simulink model "SS_continuous_ReducedObs"  (R2021a)
settings: Solver=FixedStepAuto  StartTime=0.0  StopTime=5  FixedStep=0.0001  RelTol=1e-3
values from neighbouring files (symbols this model uses):
  Ao = -1/Tm -Lc    [SS_continuous_ReducedObs_code.m]
  Bo = [km/(gbox.N*Tm), (-1/Tm -Lc)*Lc]    [SS_continuous_ReducedObs_code.m]
  Co = [0;1]    [SS_continuous_ReducedObs_code.m]
  Do = [0, 1; 0, Lc]    [SS_continuous_ReducedObs_code.m]
  K = place(F, G, p)    [SS_allDiscrete_code.m]    (also in SS_continuous_ReducedObs_code.m = place(A, B, p))
  K_robust = [Ked(2), Ked(3)]    [SS_allDiscrete_code.m]    (also in SS_continuous_ReducedObs_code.m = [Ke(2), Ke(3)])
  Ki_robust = Ked(1)    [SS_allDiscrete_code.m]    (also in SS_continuous_ReducedObs_code.m = Ke(1))
  Nu = Nxu(3)    [SS_allDiscrete_code.m]    (also in SS_continuous_ReducedObs_code.m = Nxu(3,3))
  Nx = [Nxu(1); Nxu(2)]    [SS_allDiscrete_code.m]    (also in SS_continuous_ReducedObs_code.m = [Nxu(1,3); Nxu(2,3)])
  rads2rpm = 60/2/pi    (= 9.54929658551)    [load_params_inertial_case.m]
  tauSfEst = 0.0125    [controldesign.m]
  Ts = 0.001    [SS_allDiscrete_code.m]    (also in SS_discrete_ReducedObs_code.m; discretePID_code.m)
undefined symbols (not defined in the file or in its folder): drv, gbox, mld, mot, sens
libraries: simulink x1
settings Model: Creator=giorgiadisaro  LastModifiedBy=utente-A
settings SolverCC: AlgebraicLoopSolver=TrustRegion
settings DebuggingCC: SFMachineParentedDataDiag=warning

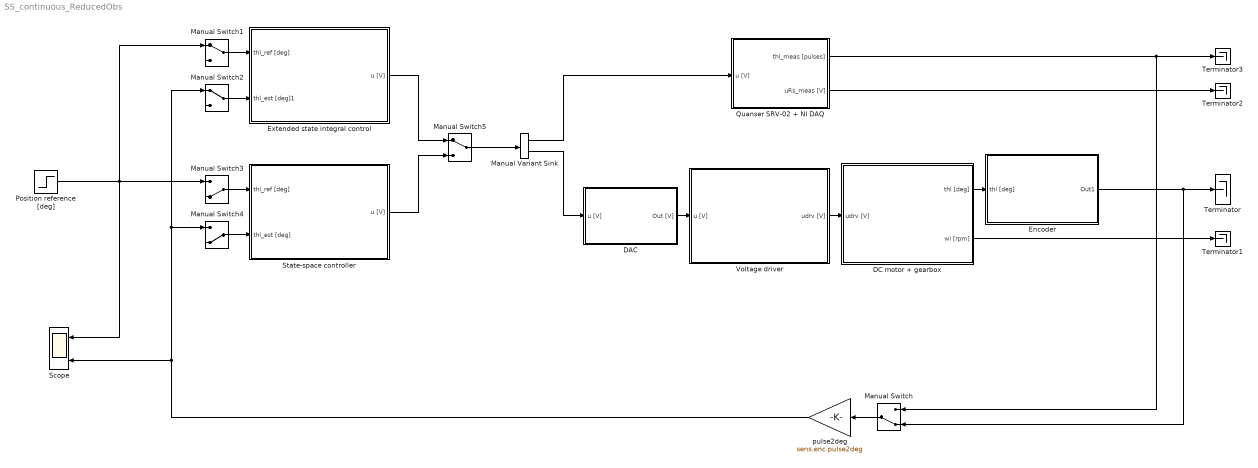
== system SS_continuous_ReducedObs ==
  DAC : Subsystem
  DC motor + gearbox : Subsystem
  Encoder : Subsystem
  Extended state integral control : Subsystem
  Manual Variant Sink : simulink/Signal Routing/Manual Variant Sink  NumChoices=2  LabelModeActiveChoice=V_2
  Manual Switch : ManualSwitch  CurrentSetting=0
  Manual Switch1 : ManualSwitch
  Manual Switch2 : ManualSwitch
  Manual Switch3 : ManualSwitch  CurrentSetting=0
  Manual Switch4 : ManualSwitch  CurrentSetting=0
  Manual Switch5 : ManualSwitch
  Position reference [deg] : Step  After=50  SampleTime=Ts
  Quanser SRV-02 + NI DAQ : Subsystem  mask(Quanser SRV-02 (with inertial load) + NI DAQ){Ts=0.001, fricType=Karnopp}
      mask prompts: Ts "NI DAQ Sample Time:"; fricType "Friction model"
      mask help: Quanser SRV-02 (with inertial load) + NI DAQ model.
      mask init:
      | %%  Sensors data
      | 
      | %   shunt resistor
      | sens.curr.Rs = 0.5;                         %   resistance [Ohm]   
      | sens.curr.uRs_std = 0.01;                   %   voltage noise standard dev [V]                           
      | sens.curr.uRs_var = sens.curr.uRs_std^2;	%   voltage noise variance [V^2]
      | 
      | %   Hewlett-Packard HEDS-5540#A06 optical encoder
      | sens.enc.ppr = 500*4;                       %   pulses per rotation
      | sens.enc.pulse2deg = 360/sens.enc.ppr;      %   [pulses] -> [deg]
      | sens.enc.pulse2rad = 2*pi/sens.enc.ppr;     %   [pulses] -> [rad]
      | sens.enc.deg2pulse = sens.enc.ppr/360;      %   [deg] -> [pulses]
      | sens.enc.rad2pulse = sens.enc.ppr/2/pi;     %   [rad] -> [pulses]
      | 
      | 
      | %%  Data acquisition board (daq) data
      | 
      | %   NI PCI-6221 DAC data
      | daq.dac.bits = 16;                                  %   resolution (bits)
      | daq.dac.fs   = 10;                                  %   full scale 
      | daq.dac.q    = 2*daq.dac.fs/(2^daq.dac.bits-1);     %	quantization
      | 
      | %   NI PCI-6221 ADC data
      | daq.adc.bits = 16;                                  %   resolution (bits)
      | daq.adc.fs   = 10;                                  %   full scale (as set in SLDRT Analog Input block)
      | daq.adc.q    = 2*daq.adc.fs/(2^daq.adc.bits-1);     %   quantization
      mask Help:
      | Riccardo Antonello (antonello@dei.unipd.it)
      | 
      | April 24, 2020
      | 
      | Dept. of Information Engineering, University of Padova
      mask TypeOptions fricType: Coulomb + viscous | Karnopp
  Scope : Scope  NumInputPorts=2
  State-space controller : Subsystem
  Terminator{,1..3} (4 alike) : Terminator
  Voltage driver : Subsystem
  pulse2deg : Gain  Gain=sens.enc.pulse2deg
  wires:
  Quanser SRV-02 + NI DAQ/2(uRs_meas [V]) -> Terminator2/1
  Manual Variant Sink/1 -> Quanser SRV-02 + NI DAQ/1(u [V])
  Manual Variant Sink/2 -> DAC/1(u [V])
  Quanser SRV-02 + NI DAQ/1(thl_meas [pulses]) -> Manual Switch/1, Terminator3/1
  DC motor + gearbox/2(wl [rpm]) -> Terminator1/1
  Manual Switch/1 -> pulse2deg/1
  DAC/1(Out [V]) -> Voltage driver/1(u [V])
  Voltage driver/1(udrv [V]) -> DC motor + gearbox/1(udrv [V])
  Position reference [deg]/1 -> Scope/1, Manual Switch1/1, Manual Switch3/1
  pulse2deg/1 -> Scope/2, Manual Switch4/1, Manual Switch2/1
  DC motor + gearbox/1("thl [deg] ") -> Encoder/1("thl [deg] ")
  Encoder/1(Out1) -> Manual Switch/2, Terminator/1
  Manual Switch1/1 -> Extended state integral control/1(thl_ref [deg])
  Manual Switch2/1 -> Extended state integral control/2(thl_est [deg]1)
  Manual Switch3/1 -> State-space controller/1(thl_ref [deg])
  Manual Switch4/1 -> State-space controller/2(thl_est [deg])
  Manual Switch5/1 -> Manual Variant Sink/1
  Extended state integral control/1(u [V]) -> Manual Switch5/1
  State-space controller/1(u [V]) -> Manual Switch5/2

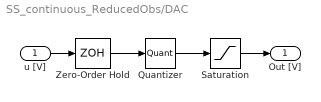
== system SS_continuous_ReducedObs/DAC ==
  u [V] : Inport
  Quantizer : Quantizer  QuantizationInterval=20/(2^16-1)
  Saturation : Saturate  UpperLimit=10  LowerLimit=-10
  Zero-Order Hold : ZeroOrderHold  SampleTime=Ts
  Out [V] : Outport
  wires:
  u [V]/1 -> Zero-Order Hold/1
  Zero-Order Hold/1 -> Quantizer/1
  Quantizer/1 -> Saturation/1
  Saturation/1 -> Out [V]/1

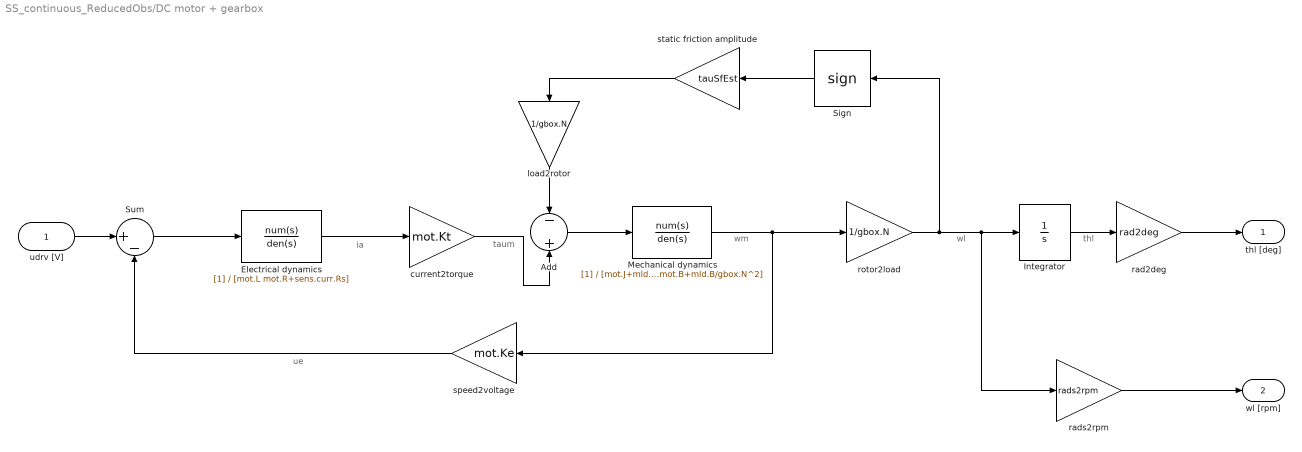
== system SS_continuous_ReducedObs/DC motor + gearbox ==
  note: thl
  note: wl
  note: wm
  note: ue
  note: taum
  note: ia
  udrv [V] : Inport
  Add : Sum  Inputs=-+
  Electrical dynamics : TransferFcn  Denominator=[mot.L mot.R+sens.curr.Rs]
  Integrator : Integrator
  Mechanical dynamics : TransferFcn  Denominator=[mot.J+mld.J/gbox.N^2 mot.B+mld.B/gbox.N^2]
  Sign : Signum  ZeroCross=off
  Sum : Sum  Inputs=|+-
  current2torque : Gain  Gain=mot.Kt
  load2rotor : Gain  Gain=1/gbox.N
  rad2deg : Gain  Gain=rad2deg
  rads2rpm : Gain  Gain=rads2rpm
  rotor2load : Gain  Gain=1/gbox.N
  speed2voltage : Gain  Gain=mot.Ke
  static friction amplitude : Gain  Gain=tauSfEst
  "thl [deg] " : Outport
  wl [rpm] : Outport  Port=2
  wires:
  static friction amplitude/1 -> load2rotor/1
  udrv [V]/1 -> Sum/1
  Electrical dynamics/1 -> current2torque/1
  current2torque/1 -> Add/2
  load2rotor/1 -> Add/1
  Sign/1 -> static friction amplitude/1
  speed2voltage/1 -> Sum/2
  rad2deg/1 -> "thl [deg] "/1
  Add/1 -> Mechanical dynamics/1
  Mechanical dynamics/1 -> speed2voltage/1, rotor2load/1
  rads2rpm/1 -> wl [rpm]/1
  Sum/1 -> Electrical dynamics/1
  rotor2load/1 -> Sign/1, rads2rpm/1, Integrator/1
  Integrator/1 -> rad2deg/1

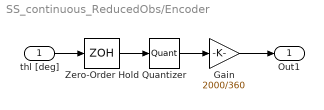
== system SS_continuous_ReducedObs/Encoder ==
  "thl [deg] " : Inport
  Gain : Gain  Gain=2000/360
  Quantizer : Quantizer  QuantizationInterval=360/(500*4)
  Zero-Order Hold : ZeroOrderHold  SampleTime=Ts
  Out1 : Outport
  wires:
  "thl [deg] "/1 -> Zero-Order Hold/1
  Zero-Order Hold/1 -> Quantizer/1
  Quantizer/1 -> Gain/1
  Gain/1 -> Out1/1

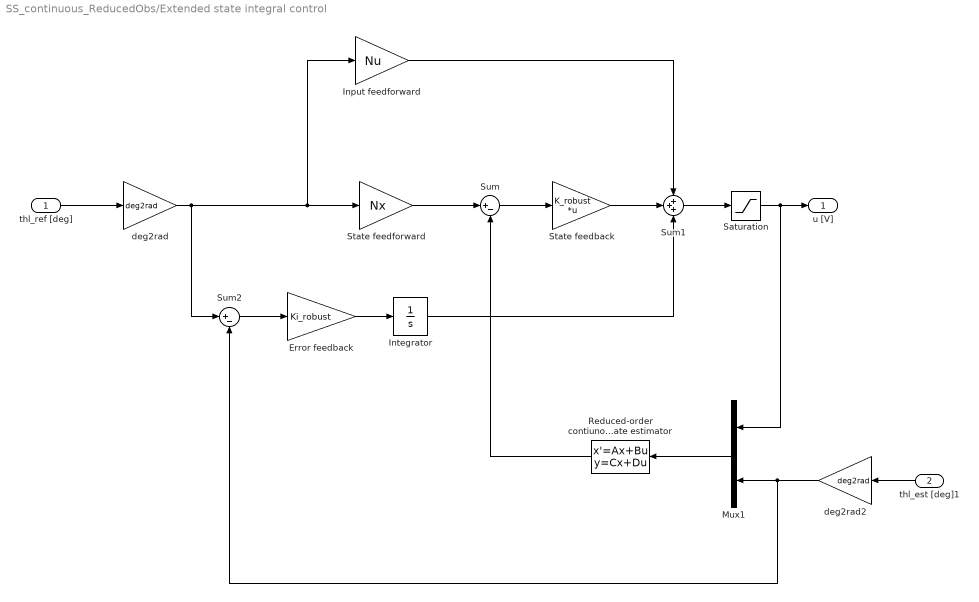
== system SS_continuous_ReducedObs/Extended state integral control ==
  thl_ref [deg] : Inport
  thl_est [deg]1 : Inport  Port=2
  Error feedback : Gain  Gain=Ki_robust
  Input feedforward : Gain  Gain=Nu
  Integrator : Integrator
  Mux1 : Mux  Inputs=2
  Reduced-order contiunous-time state estimator : StateSpace  A=Ao  B=Bo  C=Co  D=Do  InitialCondition=0
  Saturation : Saturate  UpperLimit=12  LowerLimit=-12
  State feedback : Gain  Gain=K_robust  Multiplication=Matrix(K*u)
  State feedforward : Gain  Gain=Nx
  Sum : Sum  Inputs=|+-
  Sum1 : Sum  Inputs=+++
  Sum2 : Sum  Inputs=|+-
  deg2rad : Gain  Gain=deg2rad
  deg2rad2 : Gain  Gain=deg2rad
  u [V] : Outport
  wires:
  Saturation/1 -> Mux1/1, u [V]/1
  deg2rad/1 -> State feedforward/1, Input feedforward/1, Sum2/1
  Sum/1 -> State feedback/1
  thl_ref [deg]/1 -> deg2rad/1
  State feedforward/1 -> Sum/1
  State feedback/1 -> Sum1/2
  Input feedforward/1 -> Sum1/1
  Sum1/1 -> Saturation/1
  Sum2/1 -> Error feedback/1
  Error feedback/1 -> Integrator/1
  Integrator/1 -> Sum1/3
  thl_est [deg]1/1 -> deg2rad2/1
  deg2rad2/1 -> Sum2/2, Mux1/2
  Reduced-order contiunous-time state estimator/1 -> Sum/2
  Mux1/1 -> Reduced-order contiunous-time state estimator/1

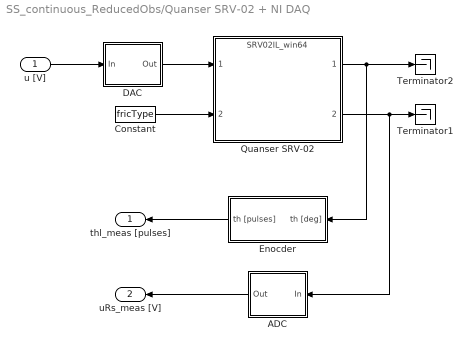
== system SS_continuous_ReducedObs/Quanser SRV-02 + NI DAQ ==
  u [V] : Inport
  ADC : Subsystem
  Constant : Constant  Value=fricType
  DAC : Subsystem
  Enocder : Subsystem
  Quanser SRV-02 : ModelReference  ModelNameDialog=SRV02IL_win64.slxp  ModelReferenceVersion=1.44  CopyOfModelProtected=on
  Terminator1 : Terminator
  Terminator2 : Terminator
  thl_meas [pulses] : Outport
  uRs_meas [V] : Outport  Port=2
  wires:
  Enocder/1(th [pulses]) -> thl_meas [pulses]/1
  ADC/1(Out) -> uRs_meas [V]/1
  DAC/1(Out) -> Quanser SRV-02/1
  Quanser SRV-02/2 -> ADC/1(In), Terminator1/1
  u [V]/1 -> DAC/1(In)
  Quanser SRV-02/1 -> Enocder/1(th [deg]), Terminator2/1
  Constant/1 -> Quanser SRV-02/2

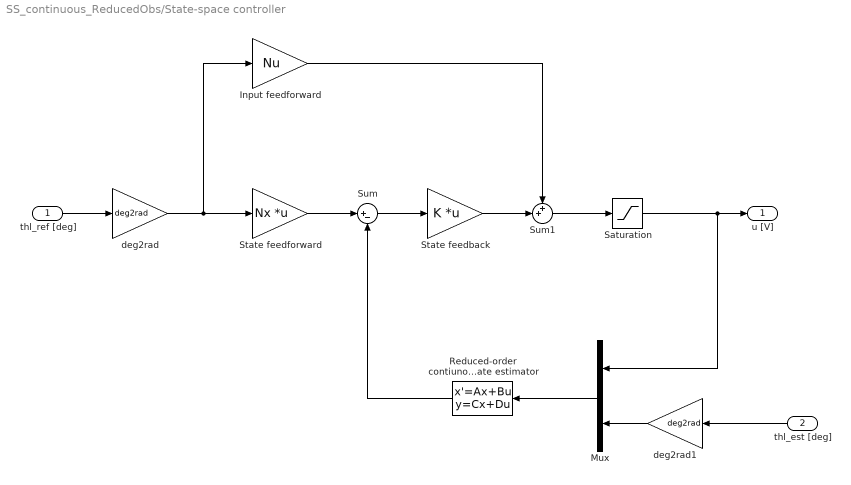
== system SS_continuous_ReducedObs/State-space controller ==
  thl_ref [deg] : Inport
  thl_est [deg] : Inport  Port=2
  Input feedforward : Gain  Gain=Nu
  Mux : Mux  Inputs=2
  Reduced-order contiunous-time state estimator : StateSpace  A=Ao  B=Bo  C=Co  D=Do  InitialCondition=0
  Saturation : Saturate  UpperLimit=12  LowerLimit=-12
  State feedback : Gain  Gain=K  Multiplication=Matrix(K*u)
  State feedforward : Gain  Gain=Nx  Multiplication=Matrix(K*u)
  Sum : Sum  Inputs=|+-
  Sum1 : Sum  Inputs=++|
  deg2rad : Gain  Gain=deg2rad
  deg2rad1 : Gain  Gain=deg2rad
  u [V] : Outport
  wires:
  Saturation/1 -> Mux/1, u [V]/1
  deg2rad/1 -> State feedforward/1, Input feedforward/1
  Sum/1 -> State feedback/1
  thl_ref [deg]/1 -> deg2rad/1
  State feedforward/1 -> Sum/1
  State feedback/1 -> Sum1/2
  Input feedforward/1 -> Sum1/1
  Sum1/1 -> Saturation/1
  thl_est [deg]/1 -> deg2rad1/1
  deg2rad1/1 -> Mux/2
  Mux/1 -> Reduced-order contiunous-time state estimator/1
  Reduced-order contiunous-time state estimator/1 -> Sum/2

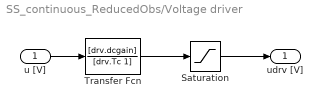
== system SS_continuous_ReducedObs/Voltage driver ==
  u [V] : Inport
  Saturation : Saturate  UpperLimit=10  LowerLimit=-10
  Transfer Fcn : TransferFcn  Numerator=[drv.dcgain]  Denominator=[drv.Tc 1]
  udrv [V] : Outport
  wires:
  u [V]/1 -> Transfer Fcn/1
  Transfer Fcn/1 -> Saturation/1
  Saturation/1 -> udrv [V]/1

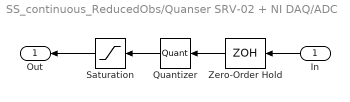
== system SS_continuous_ReducedObs/Quanser SRV-02 + NI DAQ/ADC ==
  In : Inport
  Quantizer : Quantizer  QuantizationInterval=daq.adc.q
  Saturation : Saturate  UpperLimit=daq.adc.fs  LowerLimit=-daq.adc.fs
  Zero-Order Hold : ZeroOrderHold  SampleTime=Ts
  Out : Outport
  wires:
  Saturation/1 -> Out/1
  In/1 -> Zero-Order Hold/1
  Quantizer/1 -> Saturation/1
  Zero-Order Hold/1 -> Quantizer/1

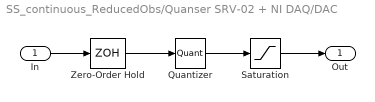
== system SS_continuous_ReducedObs/Quanser SRV-02 + NI DAQ/DAC ==
  In : Inport
  Quantizer : Quantizer  QuantizationInterval=daq.dac.q
  Saturation : Saturate  UpperLimit=daq.dac.fs  LowerLimit=-daq.dac.fs
  Zero-Order Hold : ZeroOrderHold  SampleTime=Ts
  Out : Outport
  wires:
  Quantizer/1 -> Saturation/1
  In/1 -> Zero-Order Hold/1
  Zero-Order Hold/1 -> Quantizer/1
  Saturation/1 -> Out/1

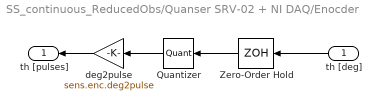
== system SS_continuous_ReducedObs/Quanser SRV-02 + NI DAQ/Enocder ==
  th [deg] : Inport
  Quantizer : Quantizer  QuantizationInterval=sens.enc.pulse2deg
  Zero-Order Hold : ZeroOrderHold  SampleTime=Ts
  deg2pulse : Gain  Gain=sens.enc.deg2pulse
  th [pulses] : Outport
  wires:
  Quantizer/1 -> deg2pulse/1
  th [deg]/1 -> Zero-Order Hold/1
  Zero-Order Hold/1 -> Quantizer/1
  deg2pulse/1 -> th [pulses]/1
